simulink model "neuron"  (R2017b)
settings: Solver=FixedStepAuto  StartTime=0.0  StopTime=100  FixedStep=0.1  RelTol=1e-3
libraries: simulink x1
settings Model: Creator=DELL  LastModifiedBy=DELL

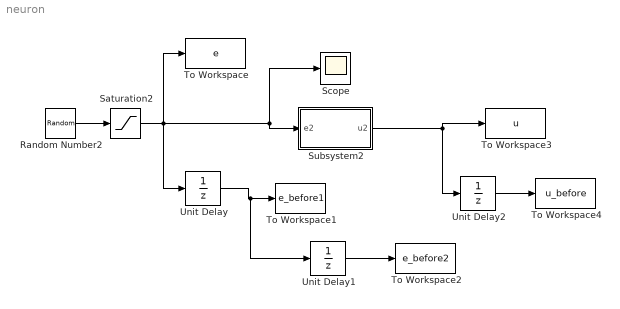
== system neuron ==
  Random Number2 : RandomNumber  Variance=200  SampleTime=0.1
  Saturation2 : Saturate  UpperLimit=0.07  LowerLimit=-0.07
  Scope : Scope
  Subsystem2 : Subsystem
  To Workspace : ToWorkspace  VariableName=e  SampleTime=-1
  To Workspace1 : ToWorkspace  VariableName=e_before1  SampleTime=-1
  To Workspace2 : ToWorkspace  VariableName=e_before2  SampleTime=-1
  To Workspace3 : ToWorkspace  VariableName=u  SampleTime=-1
  To Workspace4 : ToWorkspace  VariableName=u_before  SampleTime=-1
  Unit Delay : UnitDelay  SampleTime=-1
  Unit Delay1 : UnitDelay  SampleTime=-1
  Unit Delay2 : UnitDelay  SampleTime=-1
  wires:
  Random Number2/1 -> Saturation2/1
  Saturation2/1 -> To Workspace/1, Unit Delay/1, Subsystem2/1(e2), Scope/1
  Unit Delay1/1 -> To Workspace2/1
  Unit Delay2/1 -> To Workspace4/1
  Unit Delay/1 -> Unit Delay1/1, To Workspace1/1
  Subsystem2/1(u2) -> Unit Delay2/1, To Workspace3/1

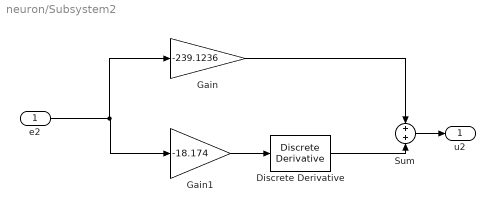
== system neuron/Subsystem2 ==
  e2 : Inport
  Discrete Derivative : simulink/Discrete/Discrete Derivative  gainval=1.0  ICPrevScaledInput=0.0  OutMin=[]  OutMax=[]  OutDataType=fixdt(1, 16)  OutScaling=2^-10  DoSatur=off
  Gain : Gain  Gain=-239.1236
  Gain1 : Gain  Gain=-18.174
  Sum : Sum
  u2 : Outport
  wires:
  Discrete Derivative/1 -> Sum/2
  Gain/1 -> Sum/1
  e2/1 -> Gain/1, Gain1/1
  Sum/1 -> u2/1
  Gain1/1 -> Discrete Derivative/1
